simulink model "CruiseControl"  (R2020b)
settings: Solver=VariableStepAuto  StartTime=0.0  StopTime=10.0  RelTol=1e-3
model workspace (MAT data in the model file):
  Kd = Simulink.Parameter
  Kd.Value = 484.0516
  Kd.DataType = 'auto'
  Kd.Dimensions = [1 1]
  Ki = Simulink.Parameter
  Ki.Value = 83.0917
  Ki.DataType = 'auto'
  Ki.Dimensions = [1 1]
  Kp = Simulink.Parameter
  Kp.Value = 495.0505
  Kp.DataType = 'auto'
  Kp.Dimensions = [1 1]
  Sig = Simulink.Signal
  Sig.DataType = 'auto'
  Sig.Dimensions = -1
  Sig.DimensionsMode = 'auto'
  Sig.Complexity = 'auto'
  Sig.SampleTime = -1
  Sig.SamplingMode = 'auto'
  Sig1 = Simulink.Signal
  Sig1.DataType = 'auto'
  Sig1.Dimensions = -1
  Sig1.DimensionsMode = 'auto'
  Sig1.Complexity = 'auto'
  Sig1.SampleTime = -1
  Sig1.SamplingMode = 'auto'
  Sig2 = Simulink.Signal
  Sig2.DataType = 'auto'
  Sig2.Dimensions = -1
  Sig2.DimensionsMode = 'auto'
  Sig2.Complexity = 'auto'
  Sig2.SampleTime = -1
  Sig2.SamplingMode = 'auto'
  Sig3 = Simulink.Signal
  Sig3.DataType = 'auto'
  Sig3.Dimensions = -1
  Sig3.DimensionsMode = 'auto'
  Sig3.Complexity = 'auto'
  Sig3.SampleTime = -1
  Sig3.SamplingMode = 'auto'
  Sig4 = Simulink.Signal
  Sig4.DataType = 'auto'
  Sig4.Dimensions = -1
  Sig4.DimensionsMode = 'auto'
  Sig4.Complexity = 'auto'
  Sig4.SampleTime = -1
  Sig4.SamplingMode = 'auto'
  Sig5 = Simulink.Signal
  Sig5.DataType = 'auto'
  Sig5.Dimensions = -1
  Sig5.DimensionsMode = 'auto'
  Sig5.Complexity = 'auto'
  Sig5.SampleTime = -1
  Sig5.SamplingMode = 'auto'
  Sig6 = Simulink.Signal
  Sig6.DataType = 'auto'
  Sig6.Dimensions = -1
  Sig6.DimensionsMode = 'auto'
  Sig6.Complexity = 'auto'
  Sig6.SampleTime = -1
  Sig6.SamplingMode = 'auto'
  Sig7 = Simulink.Signal
  Sig7.DataType = 'auto'
  Sig7.Dimensions = -1
  Sig7.DimensionsMode = 'auto'
  Sig7.Complexity = 'auto'
  Sig7.SampleTime = -1
  Sig7.SamplingMode = 'auto'
  b = Simulink.Parameter
  b.Value = 50
  b.DataType = 'auto'
  b.Dimensions = [1 1]
  m = Simulink.Parameter
  m.Value = 1000
  m.DataType = 'auto'
  m.Dimensions = [1 1]
settings Model: ParameterArgumentNames=Kd,Ki,Kp,b,m  OrderedModelArguments=off  Creator=sayali  LastModifiedBy=sayali

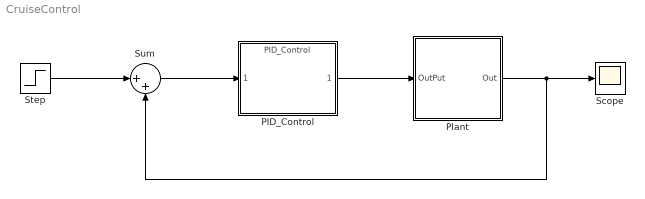
== system CruiseControl ==
  PID_Control : ModelReference  ModelNameDialog=PID_Control  UsingDefaultArgumentValue=0,0,0  SimulationMode=Normal  ModelReferenceVersion=1.6
  Plant : Subsystem
  Scope : Scope
  Step : Step  After=10  SampleTime=0
  Sum : Sum  Inputs=|++
  wires:
  PID_Control/1 -> Plant/1(OutPut)
  Plant/1(Out) -> Sum/2, Scope/1
  Step/1 -> Sum/1
  Sum/1 -> PID_Control/1

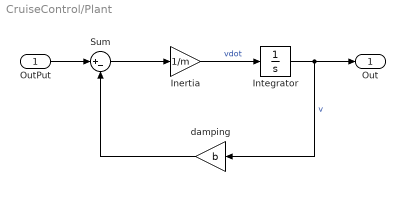
== system CruiseControl/Plant ==
  OutPut : Inport
  Inertia : Gain  Gain=1/m
  Integrator : Integrator
  Sum : Sum  Inputs=|+-
  damping : Gain  Gain=b
  Out : Outport
  wires:
  damping/1 -> Sum/2
  Sum/1 -> Inertia/1
  OutPut/1 -> Sum/1
  Integrator/1 -> Out/1, damping/1  "v"
  Inertia/1 -> Integrator/1  "vdot"
